simulink model "Test_T_Matrix_CHB_DAB"  (R2024a)
settings: Solver=ode2  StartTime=0.0  StopTime=T_end  FixedStep=Ts  RelTol=1e-3  EnableMultiTasking=on
values from neighbouring files (symbols this model uses):
  Ts = 1e-6    (= 1e-06)    [Generate_T_Matrix.m]    (also in Test_T_Matrix.m)
libraries: spsIGBTDiodeLib x12, spsSeriesRLCBranchLib x6, spsVoltageMeasurementLib x5, spsCurrentMeasurementLib x4, spsGroundLib x2, spsACVoltageSourceLib x1, spsLinearTransformerLib x1, sps_lib x1
settings Model: Creator=qy  LastModifiedBy=GAO_CX
settings SolverCC: AlgebraicLoopSolver=TrustRegion
settings DataIOCC: LimitDataPoints=on  SaveFormat=Array  SaveOutput=off  SignalLogging=off  DSMLogging=off  SaveTime=off  ReturnWorkspaceOutputs=off
settings OptimizationCC: LifeSpan=inf
settings DebuggingCC: SolverPrmCheckMsg=warning  UnconnectedInputMsg=warning  UnconnectedOutputMsg=warning  UnconnectedLineMsg=warning  SFUnexpectedBacktrackingDiag=warning  SFNoUnconditionalDefaultTransitionDiag=warning  SFExecutionAtInitializationDiag=none  ArithmeticOperatorsInVariantConditions=warning
settings HardwareCC: ProdBitPerPointer=32  ProdBitPerSizeT=32  ProdBitPerPtrDiffT=32  ProdLargestAtomicFloat=None  ProdIntDivRoundTo=Undefined  ProdEndianess=Unspecified  ProdWordSize=32  ProdHWDeviceType=32-bit Generic
settings ModelReferenceCC: PropagateSignalLabelsOutOfModel=off
settings SFSimCC: SimUseLocalCustomCode=off  CustomCodeUndefinedFunction=UseInterfaceOnly
settings RTWCC: RTWUseLocalCustomCode=off  GPUComputeCapability=3.5
settings CodeAppCC: StateflowObjectComments=on
settings GRTTargetCC: TargetLangStandard=C89/C90 (ANSI)
settings ConfigComp: CovMetricSettings=dw  CovSaveCumulativeToWorkspaceVar=on  CovSaveSingleToWorkspaceVar=on  CovExternalEMLEnable=off  CovSFcnEnable=off
settings SimscapeCC: SimscapeNormalizeSystem=off

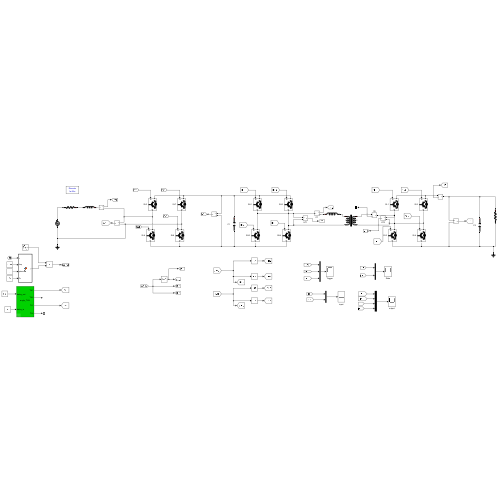
[thumbnail: Simulink's stored preview of the top-level diagram]
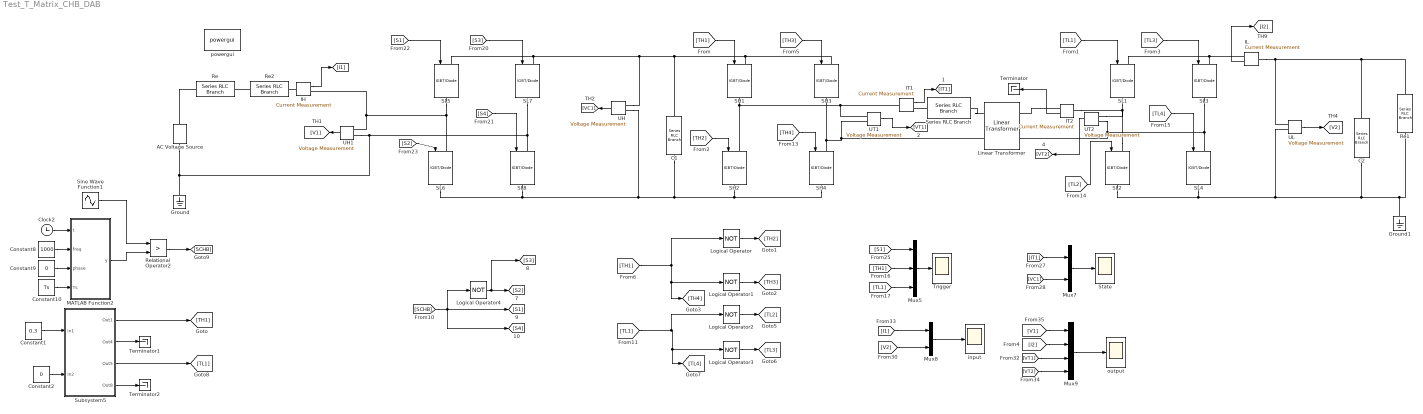
== system Test_T_Matrix_CHB_DAB ==
  AC Voltage Source : spsACVoltageSourceLib/AC Voltage Source  Amplitude=4e3  Phase=0  Frequency=50  SampleTime=0  Measurements=None  BusType=swing  Pref=10e3  Qref=0  Qmin=-inf  Qmax=+inf
  C1 : spsSeriesRLCBranchLib/Series RLC Branch  LConnTagsString=__new0  RConnTagsString=__new0  BranchType=C  Resistance=1  Inductance=1e-4  SetiL0=off  InitialCurrent=0  Capacitance=3000e-6  Setx0=off  InitialVoltage=1.5e3  Measurements=None
  C2 : spsSeriesRLCBranchLib/Series RLC Branch  LConnTagsString=__new0  RConnTagsString=__new0  BranchType=C  Resistance=1  Inductance=1e-4  SetiL0=off  InitialCurrent=0  Capacitance=1000e-6  Setx0=off  InitialVoltage=1.5e3  Measurements=None
  Clock2 : Clock
  Constant1 : Constant  Value=0.3
  Constant10 : Constant  Value=Ts
  Constant2 : Constant  Value=0
  Constant8 : Constant  Value=1000
  Constant9 : Constant  Value=0
  Ground : spsGroundLib/Ground  LConnTagsString=a
  Ground1 : spsGroundLib/Ground  LConnTagsString=a
  IH : spsCurrentMeasurementLib/Current Measurement  PhasorSimulation=off  OutputType=Complex  PSBequivalent=0
  IL : spsCurrentMeasurementLib/Current Measurement  PhasorSimulation=off  OutputType=Complex  PSBequivalent=0
  IT1 : spsCurrentMeasurementLib/Current Measurement  PhasorSimulation=off  OutputType=Complex  PSBequivalent=0
  IT2 : spsCurrentMeasurementLib/Current Measurement  PhasorSimulation=off  OutputType=Complex  PSBequivalent=0
  Linear Transformer : spsLinearTransformerLib/Linear Transformer  UNITS=pu  NominalPower=[ 0.156e6 5000 ]  winding1=[10e3 0 0]  winding2=[1e3 0 0]  ThreeWindings=off  winding3=[3.15e+05 0.002 0.08]  RmLm=[1e10 1e10]  Measurements=None  DataType=off
  Logical Operator{,1..4} (5 alike) : Logic  Operator=NOT  AllPortsSameDT=off  OutDataTypeStr=boolean
  MATLAB Function2 : MATLAB Function  TreatAsAtomicUnit=on
  Mux5 : Mux  Inputs=3
  Mux7 : Mux  Inputs=2
  Mux8 : Mux  Inputs=2
  Mux9 : Mux
  Re : spsSeriesRLCBranchLib/Series RLC Branch  LConnTagsString=__new0  RConnTagsString=__new0  BranchType=R  Resistance=0.01  Inductance=0.003  SetiL0=off  InitialCurrent=0  Capacitance=1e-6  Setx0=off  InitialVoltage=0  Measurements=None
  Re1 : spsSeriesRLCBranchLib/Series RLC Branch  LConnTagsString=__new0  RConnTagsString=__new0  BranchType=R  Resistance=1  Inductance=1e-3  SetiL0=off  InitialCurrent=0  Capacitance=1e-6  Setx0=off  InitialVoltage=0  Measurements=None
  Re2 : spsSeriesRLCBranchLib/Series RLC Branch  LConnTagsString=__new0  RConnTagsString=__new0  BranchType=L  Resistance=0.01  Inductance=0.03  SetiL0=off  InitialCurrent=0  Capacitance=1e-6  Setx0=off  InitialVoltage=0  Measurements=None
  Relational Operator2 : RelationalOperator  Operator=>  OutDataTypeStr=boolean  RndMeth=Simplest  InputSameDT=off
  SH{1..4} (4 alike) : spsIGBTDiodeLib/IGBT//Diode  Ron=1e-2  Rs=1e6  Cs=inf  Measurements=off
  SL{1..8} (8 alike) : spsIGBTDiodeLib/IGBT//Diode  Ron=1e-2  Rs=1e6  Cs=inf  Measurements=off
  Series RLC Branch : spsSeriesRLCBranchLib/Series RLC Branch  LConnTagsString=__new0  RConnTagsString=__new0  BranchType=L  Resistance=1  Inductance=0.0014  SetiL0=off  InitialCurrent=0  Capacitance=1e-6  Setx0=off  InitialVoltage=0  Measurements=None
  Sine Wave Function1 : Sin  Frequency=2*pi*50  Phase=-pi/10  SampleTime=0
  State : Scope
  Subsystem5 : Subsystem  mask(angle_TH/L){HF=5000}
      mask prompts: HF "High Frequence (HF)"
      mask help: The frequence of the transformers
      mask Display:
      | disp('angle_TH/L\n')
      | port_label('input', 1, 'delay_out')
      | port_label('input', 2, 'delay_in')
      | port_label('output', 1, 'TH1')
      | port_label('output', 2, 'TH4')
      | port_label('output', 3, 'TL1')
      | port_label('output', 4, 'TL4')
  Terminator : Terminator
  Terminator1 : Terminator
  Terminator2 : Terminator
  Trigger : Scope
  UH : spsVoltageMeasurementLib/Voltage Measurement  PhasorSimulation=off  OutputType=Complex  PSBequivalent=0
  UH1 : spsVoltageMeasurementLib/Voltage Measurement  PhasorSimulation=off  OutputType=Complex  PSBequivalent=0
  UL : spsVoltageMeasurementLib/Voltage Measurement  PhasorSimulation=off  OutputType=Complex  PSBequivalent=0
  UT1 : spsVoltageMeasurementLib/Voltage Measurement  PhasorSimulation=off  OutputType=Complex  PSBequivalent=0
  UT2 : spsVoltageMeasurementLib/Voltage Measurement  PhasorSimulation=off  OutputType=Complex  PSBequivalent=0
  input : Scope
  output : Scope
  powergui : sps_lib/powergui  Priority=1  SimulationMode=Discrete  SampleTime=Ts  frequency=60  Iterations=50  frequencyindice=0  Pbase=100e6  ErrMax=1e-4  UnitsV=kV  UnitsW=MW  buscounter=0  FunctionMessages=off  echomessages=off  EnableUseOfTLC=off  CurrentSourceSwitches=off  DisableSnubberDevices=off  DisableRonSwitches=off  DisableVfSwitches=off  DisplayEquations=off  AutomaticDiscreteSolvers=off  SolverType=Tustin  Interpol=off  ExternalGateDelay=off  methode=off  Ts=0  x0status=blocks  SPID=off  SwTol=0  HookPort=off  NonlinearTolerance=1e-4  nMaxIteration=100  ContinueOnMaxIteration=off  RestoreLinks=warning  ResistiveCurrentMeasurement=off  Frange=[0:2:500]  Ylog=off  Xlog=on  ShowGrid=off  save=off  variable=ZData  structure=0  ZoomFFT=off  StartTime=0.0  cycles=1  DisplayStyle=1  fundamental=60  FreqAxis=off  MaxFrequency=1000  frequencyindicesteady=1  RmsSteady=1  display=off
  wires:
  [TH1] -> SH1/1
  [TL1] -> SL1/1
  [TL3] -> SL3/1
  [TH3] -> SH3/1
  IH/1 -> [I1]
  UH/1 -> [VC1]
  UL/1 -> [V2]
  IL/1 -> [I2]
  IT1/1 -> [IT1]
  UT1/1 -> [VT1]
  UT2/1 -> [VT2]
  [TH2] -> SH2/1
  [TH4] -> SH4/1
  [TH1] -> Logical Operator1/1, [TH4], Logical Operator/1
  Logical Operator/1 -> [TH2]
  Logical Operator1/1 -> [TH3]
  Logical Operator2/1 -> [TL2]
  Logical Operator3/1 -> [TL3]
  [TL2] -> SL2/1
  [TL4] -> SL4/1
  Mux5/1 -> Trigger/1
  [TL1] -> [TL4], Logical Operator3/1, Logical Operator2/1
  [S2] -> SL6/1
  [S4] -> SL8/1
  [S3] -> SL7/1
  [S1] -> SL5/1
  UH1/1 -> [V1]
  [S1] -> Mux5/1
  [TH1] -> Mux5/2
  [TL1] -> Mux5/3
  Mux7/1 -> State/1
  [VC1] -> Mux7/2
  [IT1] -> Mux7/1
  Mux8/1 -> input/1
  Mux9/1 -> output/1
  [V1] -> Mux9/1
  [I2] -> Mux9/2
  [VT1] -> Mux9/3
  [I1] -> Mux8/1
  [V2] -> Mux8/2
  IT2/1 -> Terminator/1
  [VT2] -> Mux9/4
  Constant10/1 -> MATLAB Function2/4(Ts)
  Clock2/1 -> MATLAB Function2/1(t)
  MATLAB Function2/1(y) -> Relational Operator2/2
  Constant9/1 -> MATLAB Function2/3(phase)
  Constant8/1 -> MATLAB Function2/2(freq)
  Sine Wave Function1/1 -> Relational Operator2/1
  Logical Operator4/1 -> [S3], [S2]
  [SCHB] -> [S1], Logical Operator4/1, [S4]
  Relational Operator2/1 -> [SCHB]
  Subsystem5/1(Out1) -> [TH1]
  Constant2/1 -> Subsystem5/2(In2)
  Constant1/1 -> Subsystem5/1(In1)
  Subsystem5/2(Out4) -> Terminator1/1
  Subsystem5/4(Out8) -> Terminator2/1
  Subsystem5/3(Out5) -> [TL1]
  connections:
  SL1/LConn1 -- IL/RConn1 -- SL3/LConn1
  IT1/LConn1 -- SH1/RConn1 -- SH2/LConn1 -- UT1/LConn1
  SL3/RConn1 -- Linear Transformer/RConn2 -- UT2/LConn2 -- SL4/LConn1
  SL2/LConn1 -- IT2/LConn1 -- UT2/LConn1 -- SL1/RConn1
  UT1/LConn2 -- SH3/RConn1 -- SH4/LConn1 -- Linear Transformer/LConn2
  IT2/RConn1 -- Linear Transformer/RConn1
  SL8/RConn1 -- C1/RConn1 -- SH4/RConn1 -- SH2/RConn1 -- UH/LConn2 -- SL6/RConn1
  IL/LConn1 -- Re1/LConn1 -- C2/LConn1 -- UL/LConn1
  Series RLC Branch/LConn1 -- IT1/RConn1
  SL7/LConn1 -- UH/LConn1 -- SH3/LConn1 -- SH1/LConn1 -- C1/LConn1 -- SL5/LConn1
  Linear Transformer/LConn1 -- Series RLC Branch/RConn1
  SL2/RConn1 -- SL4/RConn1 -- Re1/RConn1 -- Ground1/LConn1 -- C2/RConn1 -- UL/LConn2
  AC Voltage Source/RConn1 -- Re/RConn1
  AC Voltage Source/LConn1 -- Ground/LConn1 -- UH1/LConn2 -- SL7/RConn1 -- SL8/LConn1
  SL5/RConn1 -- IH/RConn1 -- UH1/LConn1 -- SL6/LConn1
  IH/LConn1 -- Re2/LConn1
  Re2/RConn1 -- Re/LConn1

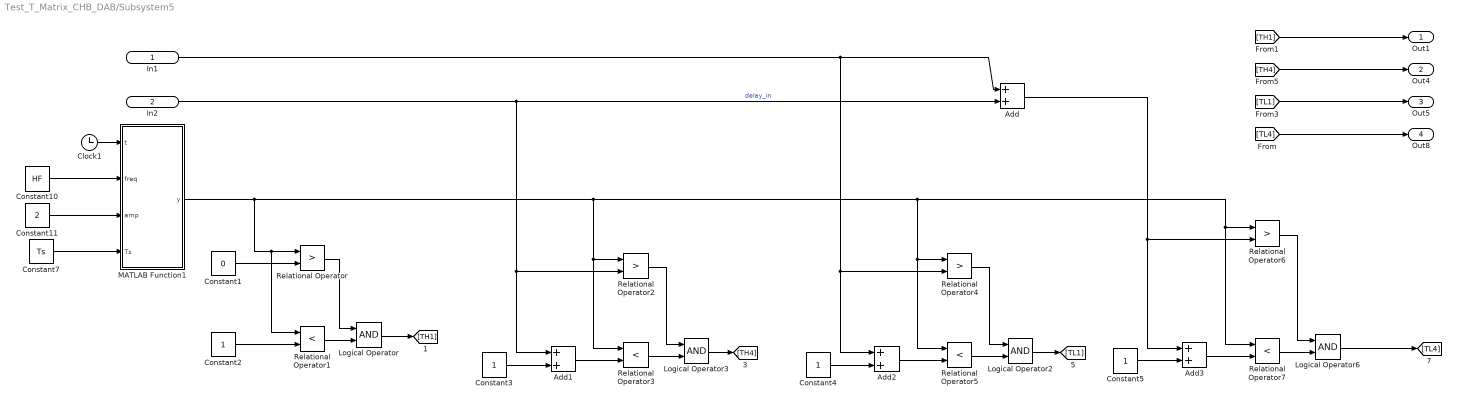
== system Test_T_Matrix_CHB_DAB/Subsystem5 ==
  In1 : Inport
  In2 : Inport  Port=2
  Add{,1..3} (4 alike) : Sum
  Clock1 : Clock
  Constant1 : Constant  Value=0
  Constant10 : Constant  Value=HF
  Constant11 : Constant  Value=2
  Constant{2..5} (4 alike) : Constant
  Constant7 : Constant  Value=Ts
  Logical Operator{,2..3,6} (4 alike) : Logic  AllPortsSameDT=off  OutDataTypeStr=boolean
  MATLAB Function1 : MATLAB Function  TreatAsAtomicUnit=on
  Relational Operator{,2,4,6} (4 alike) : RelationalOperator  Operator=>  OutDataTypeStr=boolean  RndMeth=Simplest  InputSameDT=off
  Relational Operator{1,3,5,7} (4 alike) : RelationalOperator  Operator=<  OutDataTypeStr=boolean  RndMeth=Simplest  InputSameDT=off
  Out1 : Outport
  Out4 : Outport  Port=2
  Out5 : Outport  Port=3
  Out8 : Outport  Port=4
  wires:
  [TH1] -> Out1/1
  Constant1/1 -> Relational Operator/2
  Constant2/1 -> Relational Operator1/2
  Relational Operator/1 -> Logical Operator/1
  Relational Operator1/1 -> Logical Operator/2
  In2/1 -> Relational Operator2/2, Add1/1, Add/2  "delay_in"
  Logical Operator/1 -> [TH1]
  Relational Operator2/1 -> Logical Operator3/1
  Relational Operator3/1 -> Logical Operator3/2
  Constant3/1 -> Add1/2
  Add1/1 -> Relational Operator3/2
  Logical Operator3/1 -> [TH4]
  In1/1 -> Relational Operator4/2, Add2/1, Add/1
  Add2/1 -> Relational Operator5/2
  Constant4/1 -> Add2/2
  Logical Operator2/1 -> [TL1]
  Relational Operator5/1 -> Logical Operator2/2
  Relational Operator4/1 -> Logical Operator2/1
  Add/1 -> Add3/1, Relational Operator6/2
  Add3/1 -> Relational Operator7/2
  Constant5/1 -> Add3/2
  MATLAB Function1/1(y) -> Relational Operator7/1, Relational Operator6/1, Relational Operator4/1, Relational Operator5/1, Relational Operator2/1, Relational Operator3/1, Relational Operator1/1, Relational Operator/1
  Logical Operator6/1 -> [TL4]
  Relational Operator7/1 -> Logical Operator6/2
  Relational Operator6/1 -> Logical Operator6/1
  [TH4] -> Out4/1
  [TL4] -> Out8/1
  [TL1] -> Out5/1
  Constant10/1 -> MATLAB Function1/2(freq)
  Clock1/1 -> MATLAB Function1/1(t)
  Constant7/1 -> MATLAB Function1/4(Ts)
  Constant11/1 -> MATLAB Function1/3(amp)

== matlab function Test_T_Matrix_CHB_DAB/Subsystem5/MATLAB Function1 ==
  data: t input; y output; freq input; amp input; Ts input
function y = triangle_wave(t,freq, amp,Ts)
       
    T=1.0/freq;
    tot_num=T/Ts;
    
    t_period=mod(t,T);
    count=round(t_period/Ts);

    step=amp/(tot_num);    
    if(abs(count-0)<1e-3)
        y=1e-3;
    else
        y=count*step;
    end
    
end

== matlab function Test_T_Matrix_CHB_DAB/MATLAB Function2 ==
  data: t input; y output; freq input; phase input; Ts input
function y= Tri(t,freq, phase, Ts)
    amp=1;
    T=1.0/freq;
    phase_time = phase / 360 * T; % 相位转换为时间
    tot_num = round(T / Ts);
    step=2*amp/(T/Ts/2);
    
    t_period=mod(t+phase_time,T);
    count_period=round(t_period/Ts);

    if(count_period<=tot_num/2)
        y=-amp+count_period*step;
    else
        y=(tot_num-count_period)*step-amp;
    end
end
